simulink subsystem "PvtSubSys_VSM_ESS"  (R2020b)
settings: Solver=VariableStepAuto  StartTime=0.0  StopTime=10.0  RelTol=1e-3
values from neighbouring files (symbols this model uses):
  P_VSM_ESS_AccelPed_enable = 1.0    [ESS.sldd]
  P_VSM_ESS_AccPedlPosn_Param = 60.0    [ESS.sldd]
  P_VSM_ESS_ACtiveTime = 5.0    [ESS.sldd]
  P_VSM_ESS_AEBFlag_enable = 1.0    [ESS.sldd]
  P_VSM_ESS_AngleSpdTable_deg : value not decoded    [ESS.sldd]
  P_VSM_ESS_DangerPlausLeft = 0.3    [ESS.sldd]
  P_VSM_ESS_DangerPlausRight = 0.3    [ESS.sldd]
  P_VSM_ESS_DelayTime = 3.0    [ESS.sldd]
  P_VSM_ESS_DoorSts_enable = 1.0    [ESS.sldd]
  P_VSM_ESS_DriveIn : value not decoded    [ESS.sldd]
  P_VSM_ESS_DriveIn_BP : value not decoded    [ESS.sldd]
  P_VSM_ESS_DriverInputdSameDire_delaytime = 1.0    [ESS.sldd]
  P_VSM_ESS_DriverInputTrq_Param : value not decoded    [ESS.sldd]
  P_VSM_ESS_DrvOverTime_Param = 0.2    [ESS.sldd]
  P_VSM_ESS_DrvOverTime_Paramsame = 0.2    [ESS.sldd]
  P_VSM_ESS_DrvSBR_enable = 1.0    [ESS.sldd]
  P_VSM_ESS_ESPActive_enable = 1.0    [ESS.sldd]
  P_VSM_ESS_ESPFuncOffSts_enable = 1.0    [ESS.sldd]
  P_VSM_ESS_FcwDisFlag_enable = 1.0    [ESS.sldd]
  P_VSM_ESS_FcwSw_enable = 1.0    [ESS.sldd]
  P_VSM_ESS_HiLoBeam_enable = 1.0    [ESS.sldd]
  P_VSM_ESS_IPSpeed_kmh : value not decoded    [ESS.sldd]
  P_VSM_ESS_LateralAccel_enable = 1.0    [ESS.sldd]
  P_VSM_ESS_LgtAccelLower_Param = -8.0    [ESS.sldd]
  P_VSM_ESS_LgtAccelUpper_Param = 3.0    [ESS.sldd]
  P_VSM_ESS_MasterCylindBrake = 5.0    [ESS.sldd]
  P_VSM_ESS_MaxLateral_mss : value not decoded    [ESS.sldd]
  P_VSM_ESS_OVERRIDE_SW = 0.0    [ESS.sldd]
  P_VSM_ESS_SafeDistance_m = 1.5    [ESS.sldd]
  P_VSM_ESS_SpdPoint_kmh : value not decoded    [ESS.sldd]
  P_VSM_ESS_SpdTime_s : value not decoded    [ESS.sldd]
  P_VSM_ESS_SteerWheelSpd_BP : value not decoded    [ESS.sldd]
  P_VSM_ESS_SteerWheelSpd_enable = 1.0    [ESS.sldd]
  P_VSM_ESS_SteerWheelSpd_Param : value not decoded    [ESS.sldd]
  P_VSM_ESS_StopA0_Param = 0.2    [ESS.sldd]
  P_VSM_ESS_StopA1_Param = 0.02    [ESS.sldd]
  P_VSM_ESS_StopA1Time_Param = 2.0    [ESS.sldd]
  P_VSM_ESS_TrailerSts_enable = 1.0    [ESS.sldd]
  P_VSM_ESS_VehLgtAccel_enable = 1.0    [ESS.sldd]
  P_VSM_ESS_Vehspeed_enable = 1.0    [ESS.sldd]
  P_VSM_ESS_WiprReq_enable = 1.0    [ESS.sldd]
undefined symbols (not defined in the file or in its folder): P_Global_WheelBase_m
libraries: simulink x104, TrueDurationTime x6
(part 3 of 3)

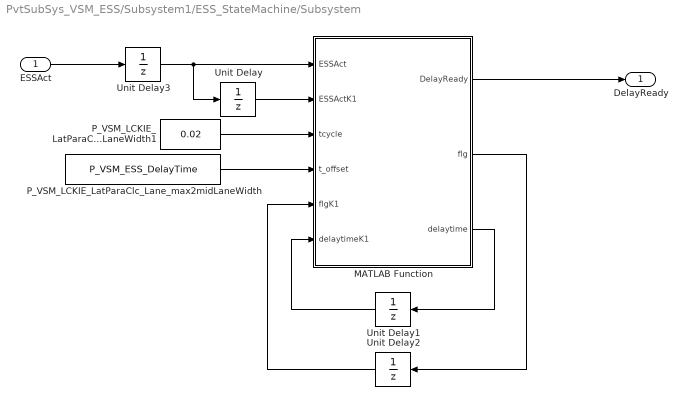
== system PvtSubSys_VSM_ESS/Subsystem1/ESS_StateMachine/Subsystem ==
  ESSAct : Inport
  MATLAB Function : MATLAB Function  TreatAsAtomicUnit=on
  P_VSM_LCKIE_LatParaClc_Lane_max2midLaneWidth : Constant  Value=P_VSM_ESS_DelayTime
  P_VSM_LCKIE_LatParaClc_Lane_max2midLaneWidth1 : Constant  Value=0.02  OutDataTypeStr=single
  Unit Delay{,1..3} (4 alike) : UnitDelay  SampleTime=-1  HasFrameUpgradeWarning=on
  DelayReady : Outport
  wires:
  ESSAct/1 -> Unit Delay3/1
  Unit Delay/1 -> MATLAB Function/2(ESSActK1)
  MATLAB Function/2(flg) -> Unit Delay2/1
  P_VSM_LCKIE_LatParaClc_Lane_max2midLaneWidth1/1 -> MATLAB Function/3(tcycle)
  P_VSM_LCKIE_LatParaClc_Lane_max2midLaneWidth/1 -> MATLAB Function/4(t_offset)
  Unit Delay1/1 -> MATLAB Function/6(delaytimeK1)
  MATLAB Function/3(delaytime) -> Unit Delay1/1
  Unit Delay2/1 -> MATLAB Function/5(flgK1)
  MATLAB Function/1(DelayReady) -> DelayReady/1
  Unit Delay3/1 -> Unit Delay/1, MATLAB Function/1(ESSAct)

== matlab function PvtSubSys_VSM_ESS/Subsystem1/ESS_StateMachine/ESS_Condition/MATLAB Function ==
  data: u input; y output; fgk1 input; ck1 input; fg output; c output
function [y,fg,c]= fcn(u,fgk1,ck1)
y=false;
fg=0;
c=0;
if u>0 
    fg=1;
    y=true;
end
if fgk1>0 && u==0
    c=ck1+1;
    fg=1;
    y=true;
end
if ck1>50
    y=false;
    fg=0;
    c=0;
end

== matlab function PvtSubSys_VSM_ESS/Subsystem1/ESS_StateMachine/ESS_Condition/MATLAB Function1 ==
  data: LgAcc input; y output; uper input; lower input
function y = fcn(LgAcc,uper,lower)
y=0;
if LgAcc<uper && LgAcc>lower
    y=1;
end

== stateflow chart PvtSubSys_VSM_ESS/Subsystem1/ESS_StateMachine/ESS_State ==
  settings: executeAtInitialization=1
  state MAINST_ERROR
    en:ESS_STATE = 6;
  state MAINST_OFF
    en:ESS_STATE = 0;
  state MAINST_ON
    state SUBST_IDLE
      en:ESS_STATE = 1;
    state SUBST_READY
      en:ESS_STATE = 2;
    state SUB_ACTIVE
      %en:ESS_STATE = 3;
      state SUB_ACTIVE_LEFT
        en:ESS_STATE = 4;L=uint16(0);
        during:L = L + uint16(1);
      state SUB_ACTIVE_RIGHT
        en:ESS_STATE = 5;R=uint16(0);
        during:R = R + uint16(1);
      state ACT
        en:ESS_STATE = 2;
      (default) -> ACT
      ACT -> SUB_ACTIVE_LEFT [order 2] : [ESS_LEFT_READY2ACTIVE]
      ACT -> SUB_ACTIVE_RIGHT [order 1] : [ESS_RIGHT_READY2ACTIVE]
    (default) -> SUBST_IDLE
    SUB_ACTIVE -> SUBST_IDLE : [ESS_ACTIVE2IDLE]
    SUBST_IDLE -> SUBST_READY : [ESS_IDLE2READY]
    SUBST_READY -> SUBST_IDLE [order 1] : [ESS_READY2IDLE]
    SUB_ACTIVE_LEFT -> SUBST_READY : [ESS_L_ACTIVE2READY||L>ESS_ACtime]{L=uint16(0);}
    SUBST_READY -> SUB_ACTIVE [order 2] : [ESS_READY2ACTIVE&&delaytime]
    SUB_ACTIVE_RIGHT -> SUBST_READY : [ESS_R_ACTIVE2READY||R>ESS_ACtime]{R=uint16(0);}
  (default) -> MAINST_OFF
  MAINST_ERROR -> MAINST_OFF [order 1] : [(ESS_PedSwtReq==false&&...
      | ESS_VehSwtReq==false)||VehConfigESS==0]
  MAINST_OFF -> MAINST_ERROR [order 1] : [(ESS_PedSwtReq==true||ESS_VehSwtReq==true)&&...
      | ERROR==true&&VehConfigESS==1]
  MAINST_OFF -> MAINST_ON [order 2] : [(ESS_PedSwtReq==true||...
      | ESS_VehSwtReq==true)&&ERROR==false&&...
      | VehConfigESS==1]
  MAINST_ON -> MAINST_OFF [order 1] : [(ESS_PedSwtReq==false&&...
      | ESS_VehSwtReq==false)||VehConfigESS==0]
  MAINST_ERROR -> MAINST_ON [order 2] : [ERROR==false]
  MAINST_ON -> MAINST_ERROR [order 2] : [ERROR==true]
  data: ESS_PedSwtReq input boolean size=1; ESS_VehSwtReq input boolean size=1; ERROR input boolean size=1; ESS_IDLE2READY input boolean size=1; ESS_READY2IDLE input boolean size=1; ESS_READY2ACTIVE input boolean size=1; ESS_ACTIVE2IDLE input boolean size=1; ESS_STATE output uint8 size=1; ESS_L_ACTIVE2READY input boolean size=1; ESS_R_ACTIVE2READY input boolean size=1; ESS_LEFT_READY2ACTIVE input boolean size=1; ESS_RIGHT_READY2ACTIVE input boolean size=1; VehConfigESS input uint8; ESS_ACtime input single; R output uint16; L output uint16; delaytime input boolean

== matlab function PvtSubSys_VSM_ESS/Subsystem1/ESS_StateMachine/FCWObjExist ==
  data: FCWObjExist output boolean size=1; FCWObjID input uint8 size=1; ESS_act_ID output uint8 size=1; pre_FCWObjID input uint8 size=1; pre_ESS_act_ID input uint8 size=1; pre_counter input uint8 size=1; counter output uint8 size=1
function [FCWObjExist,ESS_act_ID,counter] = fcn(FCWObjID,pre_FCWObjID,pre_ESS_act_ID,pre_counter)
ESS_act_ID = pre_ESS_act_ID;
counter = pre_counter;
if FCWObjID ~= 0 && pre_FCWObjID == 0
    ESS_act_ID = FCWObjID;
    counter = uint8(0);
end
if FCWObjID ~= ESS_act_ID
    counter = counter + 1;
end
if counter >= 2500
    FCWObjExist = false;
else
    FCWObjExist = true;
end

== matlab function PvtSubSys_VSM_ESS/Subsystem1/ESS_StateMachine/MATLAB Function4 ==
  data: angle input; t input; Dmin output; L input; Tx output; V input; d input; D output
function [Dmin,Tx,D] = fcn(angle,t,L,V,d)
R=V/angle;% t : reaction time; angle: runing max angle;
S=sqrt(R^2-(R-(L*0.5))^2);
Tx=S/V;
D= Tx*1*V;
Dmin= Tx*1.2*V+V*t+d; % d: static safe distance;

== matlab function PvtSubSys_VSM_ESS/Subsystem1/ESS_StateMachine/Subsystem/MATLAB Function ==
  data: DelayReady output boolean; ESSAct input boolean; flg output uint8; ESSActK1 input boolean; tcycle input single; t_offset input single; flgK1 input uint8; delaytimeK1 input single; delaytime output single
function [DelayReady,flg,delaytime] = fcn(ESSAct,ESSActK1,tcycle,t_offset,flgK1,delaytimeK1)

flg = uint8(0);
delaytime = single(0);
DelayReady = true;


if ESSAct==0 && ESSActK1==1
    flg = uint8(1);
    delaytime = tcycle;
    DelayReady = false;
end
if flgK1==1
    delaytime = delaytimeK1 + tcycle;
    if delaytime < t_offset
        flg = uint8(1);
        DelayReady = false;
    end
end
